simulink model "f3"  (R2021b)
settings: Solver=FixedStepAuto  StartTime=0.0  StopTime=10.0  RelTol=1e-3
libraries: simulink x4
settings Model: Creator=asus  LastModifiedBy=asus

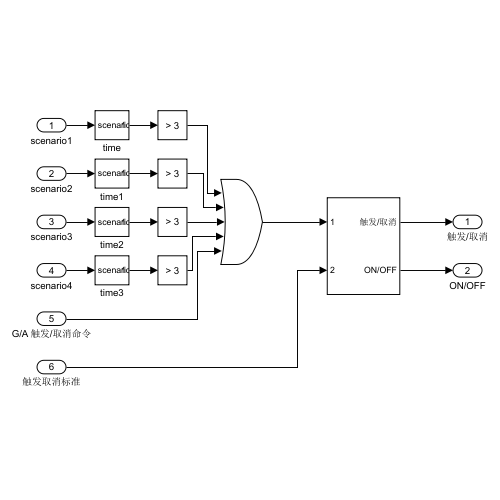
[thumbnail: Simulink's stored preview of the top-level diagram]
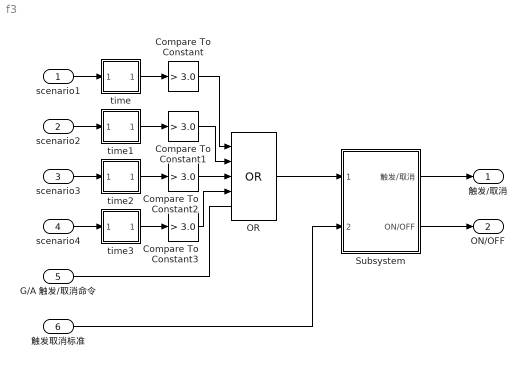
== system f3 ==
  scenario1 : Inport
  scenario2 : Inport  Port=2
  scenario3 : Inport  Port=3
  scenario4 : Inport  Port=4
  G/A 触发/取消命令 : Inport  Port=5
  触发取消标准 : Inport  Port=6
  Compare To Constant{,1..3} (4 alike) : simulink/Logic and Bit Operations/Compare To Constant  relop=>  const=3.0  OutDataTypeStr=boolean
  OR : Logic  Operator=OR  Inputs=5  IconShape=distinctive  AllPortsSameDT=off  OutDataTypeStr=boolean
  Subsystem : Subsystem
  time : Subsystem
  time1 : Subsystem
  time2 : Subsystem
  time3 : Subsystem
  触发/取消 : Outport
  ON/OFF : Outport  Port=2
  wires:
  G/A 触发/取消命令/1 -> OR/5
  scenario1/1 -> time/1(scenario1)
  scenario2/1 -> time1/1(scenario2)
  scenario3/1 -> time2/1(scenario3)
  scenario4/1 -> time3/1(scenario4)
  time/1(Out1) -> Compare To Constant/1
  time1/1(Out1) -> Compare To Constant1/1
  time2/1(Out1) -> Compare To Constant2/1
  time3/1(Out1) -> Compare To Constant3/1
  Compare To Constant2/1 -> OR/3
  Compare To Constant1/1 -> OR/2
  Compare To Constant3/1 -> OR/4
  Compare To Constant/1 -> OR/1
  OR/1 -> Subsystem/1(1)
  触发取消标准/1 -> Subsystem/2(2)
  Subsystem/1(触发/取消) -> 触发/取消/1
  Subsystem/2(ON/OFF) -> ON/OFF/1

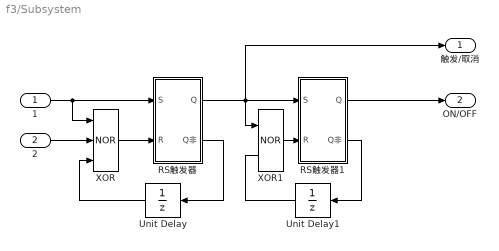
== system f3/Subsystem ==
  1 : Inport
  2 : Inport  Port=2
  RS触发器 : Subsystem
  RS触发器1 : Subsystem
  Unit Delay : UnitDelay  SampleTime=-1  HasFrameUpgradeWarning=on
  Unit Delay1 : UnitDelay  SampleTime=-1  HasFrameUpgradeWarning=on
  XOR : Logic  Operator=NOR  Inputs=3  IconShape=distinctive  AllPortsSameDT=off  OutDataTypeStr=boolean
  XOR1 : Logic  Operator=NOR  IconShape=distinctive  AllPortsSameDT=off  OutDataTypeStr=boolean
  触发/取消 : Outport
  ON/OFF : Outport  Port=2
  wires:
  1/1 -> XOR/1, RS触发器/1(S)
  RS触发器1/2(Q非) -> Unit Delay1/1
  XOR/1 -> RS触发器/2(R)
  XOR1/1 -> RS触发器1/2(R)
  Unit Delay/1 -> XOR/3
  RS触发器/1(Q) -> 触发/取消/1, XOR1/1, RS触发器1/1(S)
  Unit Delay1/1 -> XOR1/2
  RS触发器/2(Q非) -> Unit Delay/1
  2/1 -> XOR/2
  RS触发器1/1(Q) -> ON/OFF/1

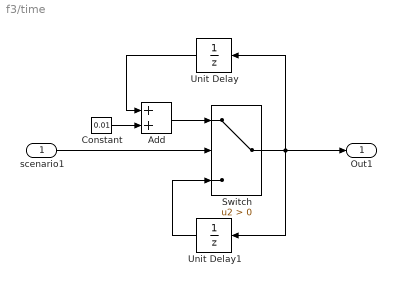
== system f3/time ==
  scenario1 : Inport
  Add : Sum
  Constant : Constant  Value=0.01
  Switch : Switch  Criteria=u2 > Threshold
  Unit Delay : UnitDelay  SampleTime=-1  HasFrameUpgradeWarning=on
  Unit Delay1 : UnitDelay  SampleTime=-1  HasFrameUpgradeWarning=on
  Out1 : Outport
  wires:
  scenario1/1 -> Switch/2
  Unit Delay/1 -> Add/1
  Switch/1 -> Out1/1, Unit Delay/1, Unit Delay1/1
  Constant/1 -> Add/2
  Add/1 -> Switch/1
  Unit Delay1/1 -> Switch/3

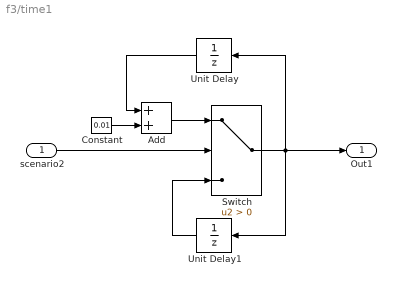
== system f3/time1 ==
  scenario2 : Inport
  Add : Sum
  Constant : Constant  Value=0.01
  Switch : Switch  Criteria=u2 > Threshold
  Unit Delay : UnitDelay  SampleTime=-1  HasFrameUpgradeWarning=on
  Unit Delay1 : UnitDelay  SampleTime=-1  HasFrameUpgradeWarning=on
  Out1 : Outport
  wires:
  Unit Delay1/1 -> Switch/3
  Add/1 -> Switch/1
  Constant/1 -> Add/2
  Switch/1 -> Unit Delay1/1, Unit Delay/1, Out1/1
  Unit Delay/1 -> Add/1
  scenario2/1 -> Switch/2

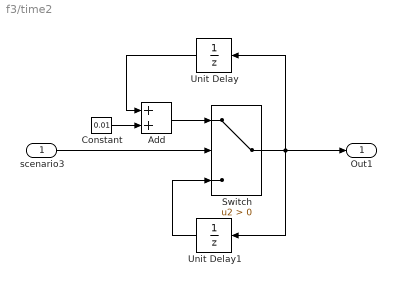
== system f3/time2 ==
  scenario3 : Inport
  Add : Sum
  Constant : Constant  Value=0.01
  Switch : Switch  Criteria=u2 > Threshold
  Unit Delay : UnitDelay  SampleTime=-1  HasFrameUpgradeWarning=on
  Unit Delay1 : UnitDelay  SampleTime=-1  HasFrameUpgradeWarning=on
  Out1 : Outport
  wires:
  Unit Delay1/1 -> Switch/3
  Add/1 -> Switch/1
  Constant/1 -> Add/2
  Switch/1 -> Unit Delay1/1, Unit Delay/1, Out1/1
  Unit Delay/1 -> Add/1
  scenario3/1 -> Switch/2

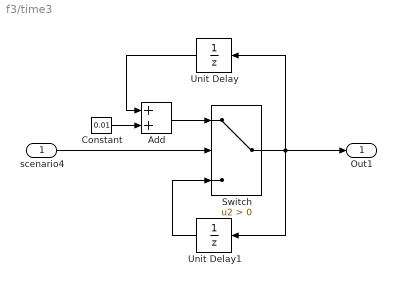
== system f3/time3 ==
  scenario4 : Inport
  Add : Sum
  Constant : Constant  Value=0.01
  Switch : Switch  Criteria=u2 > Threshold
  Unit Delay : UnitDelay  SampleTime=-1  HasFrameUpgradeWarning=on
  Unit Delay1 : UnitDelay  SampleTime=-1  HasFrameUpgradeWarning=on
  Out1 : Outport
  wires:
  scenario4/1 -> Switch/2
  Unit Delay/1 -> Add/1
  Switch/1 -> Out1/1, Unit Delay/1, Unit Delay1/1
  Constant/1 -> Add/2
  Add/1 -> Switch/1
  Unit Delay1/1 -> Switch/3

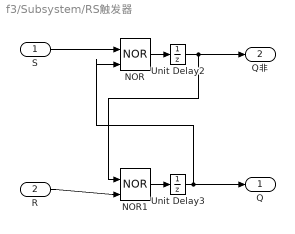
== system f3/Subsystem/RS触发器 ==
  S : Inport
  R : Inport  Port=2
  NOR : Logic  Operator=NOR  IconShape=distinctive  AllPortsSameDT=off  OutDataTypeStr=boolean
  NOR1 : Logic  Operator=NOR  IconShape=distinctive  AllPortsSameDT=off  OutDataTypeStr=boolean
  Unit Delay2 : UnitDelay  SampleTime=-1  HasFrameUpgradeWarning=on
  Unit Delay3 : UnitDelay  SampleTime=-1  HasFrameUpgradeWarning=on
  Q : Outport
  Q非 : Outport  Port=2
  wires:
  S/1 -> NOR/1
  R/1 -> NOR1/2
  NOR1/1 -> Unit Delay3/1
  NOR/1 -> Unit Delay2/1
  Unit Delay2/1 -> NOR1/1, Q非/1
  Unit Delay3/1 -> NOR/2, Q/1

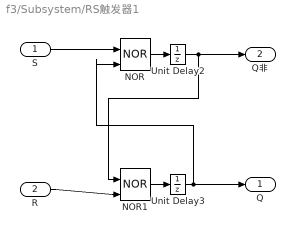
== system f3/Subsystem/RS触发器1 ==
  S : Inport
  R : Inport  Port=2
  NOR : Logic  Operator=NOR  IconShape=distinctive  AllPortsSameDT=off  OutDataTypeStr=boolean
  NOR1 : Logic  Operator=NOR  IconShape=distinctive  AllPortsSameDT=off  OutDataTypeStr=boolean
  Unit Delay2 : UnitDelay  SampleTime=-1  HasFrameUpgradeWarning=on
  Unit Delay3 : UnitDelay  SampleTime=-1  HasFrameUpgradeWarning=on
  Q : Outport
  Q非 : Outport  Port=2
  wires:
  Unit Delay3/1 -> Q/1, NOR/2
  Unit Delay2/1 -> Q非/1, NOR1/1
  NOR/1 -> Unit Delay2/1
  NOR1/1 -> Unit Delay3/1
  R/1 -> NOR1/2
  S/1 -> NOR/1
